simulink model "aeb_rzr"  (R2023b)
settings: Solver=FixedStepAuto  StartTime=0.0  StopTime=inf  RelTol=1e-3
undefined symbols (not defined in the file): camera, gray
libraries: visionanalysis x1, visiongeotforms x1
CloseFcn:
  | helperSLVisionVehicleDetectorCleanUp
settings Model: SILPILSystemUnderTest=refmodels  Creator=The MathWorks, Inc.  LastModifiedBy=tsamak
settings SolverCC: AlgebraicLoopSolver=TrustRegion  MaxZcPerStep=1
settings DataIOCC: SaveFormat=StructureWithTime  SaveOutput=off  DSMLogging=off  SaveTime=off
settings OptimizationCC: DefaultParameterBehavior=Inlined  EnhancedBackFolding=on  PassReuseOutputArgsThreshold=0  ZeroExternalMemoryAtStartup=off  ZeroInternalMemoryAtStartup=off  InitFltsAndDblsToZero=on  OptimizeBlockOrder=speed  DifferentSizesBufferReuse=on  OptimizationCustomize=off
settings DebuggingCC: ParameterTunabilityLossMsg=error  UnconnectedInputMsg=warning  UnconnectedOutputMsg=warning  UnconnectedLineMsg=warning  SubsystemReferenceDiagnosticForUnitTest=warning
settings HardwareCC: ProdLongLongMode=on  TargetLongLongMode=on
settings ModelReferenceCC: EnableRefExpFcnMdlSchedulingChecks=on
settings SFSimCC: SimTargetLang=C++
settings RTWCC: CodeExecutionProfiling=on  CodeProfilingSaveOptions=AllData  TargetLang=C++  GenerateGPUCode=CUDA  DLArmComputeVersion=19.05
settings CodeAppCC: ForceParamTrailComments=on  OperatorAnnotations=on
settings GRTTargetCC: TargetLangStandard=C++11 (ISO)  CodeInterfacePackaging=C++ class
settings ConfigComp: CovScope=ReferencedModels  CovIncludeTopModel=off  CovExternalEMLEnable=off  CovSFcnEnable=off

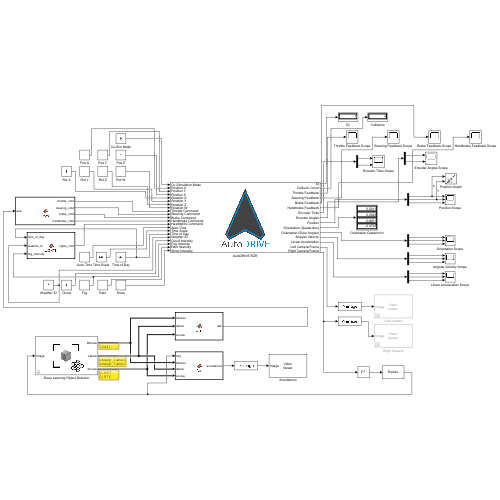
[thumbnail: Simulink's stored preview of the top-level diagram]
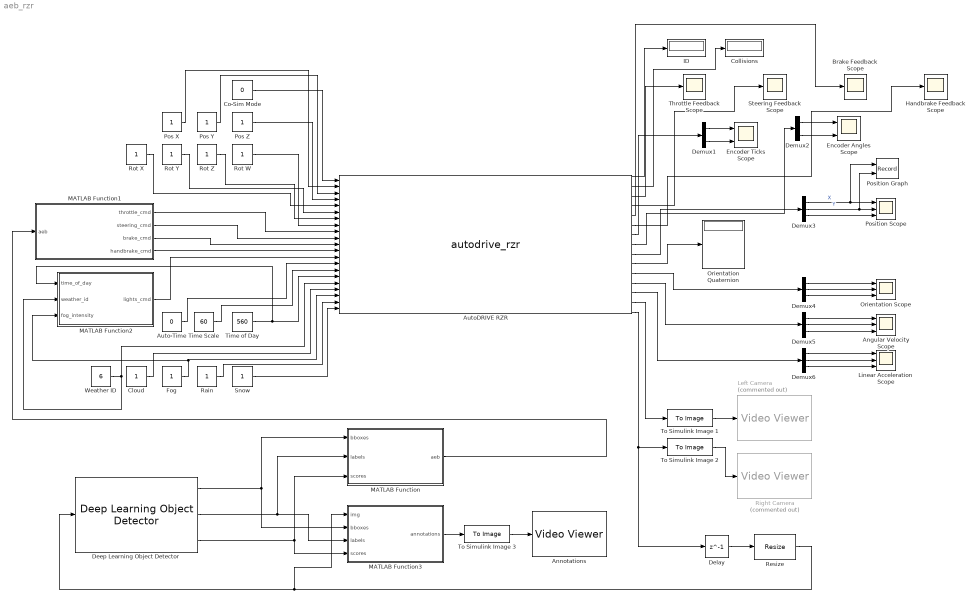
== system aeb_rzr ==
  Angular Velocity Scope : Scope  NumInputPorts=3
  Annotations : VideoViewer  colormapValue=gray(256)  FigPos=[1241.66666666667 442 408 253.333333333333]
  Auto-Time : Constant  Value=0  OutDataTypeStr=boolean
  AutoDRIVE RZR : M-S-Function  FunctionName=autodrive_rzr  Parameters=Port  mask{Port=4567}
      mask Display:
      | image('autodrive_logo.png');
      | port_label('input', 1, 'Co-Simulation Mode');
      | port_label('input', 2, 'Position X');
      | port_label('input', 3, 'Position Y');
      | port_label('input', 4, 'Position Z');
      | port_label('input', 5, 'Rotation X');
      | port_label('input', 6, 'Rotation Y');
      | port_label('input', 7, 'Rotation Z');
      | port_label('input', 8, 'Rotation W');
      | port_label('input', 9, 'Throttle Command');
      | port_label('input', 10, 'Steering Command');
      | port_label('input', 11, 'Brake Command');
      | port_label('input', 12, 'Handbrake Command');
      | port_label('input', 13, 'Headlights Command');
      | port_label('input', 14, 'Auto-Time');
      | port_label('input', 15, 'Time Scale');
      | port_label('input', 16, 'Time of Day');
      | port_label('input', 17, 'Weather ID');
      | port_label('input', 18, 'Cloud Intensity');
      | port_label('input', 19, 'Fog Intensity');
      | port_label('input', 20, 'Rain Intensity');
      | port_label('input', 21, 'Snow Intensity');
      | port_label('output', 1, 'ID');
      | port_label('output', 2, 'Collision Count');
      | port_label('output', 3, 'Throttle Feedback');
      | port_label('output', 4, 'Steering Feedback');
      | port_label('output', 5, 'Brake Feedback');
      | port_label('output', 6, 'Handbrake Feedback');
      | port_label('output', 7, 'Encoder Ticks');
      | port_label('output', 8, 'Encoder Angles');
      | port_label('output', 9, 'Position');
      | port_label('output', 10, 'Orientation (Quaternion)');
      | port_label('output', 11, 'Orientation (Euler Angles)');
      | port_label('output', 12, 'Angular Velocity');
      | port_label('output', 13, 'Linear Acceleration');
      | port_label('output', 14, 'Left Camera Frame');
      | port_label('output', 15, 'Right Camera Frame');
  Brake Feedback Scope : Scope
  Cloud : Constant
  Co-Sim Mode : Constant  Value=0  OutDataTypeStr=uint8
  Collisions : Display
  Deep Learning Object Detector : visionanalysis/Deep Learning Object Detector  Detector=Detector from MAT-file  DetectorFunction=vehicleDetectorYOLOv2  DetectorFilePath=C:\Users\tsamak\Downloads\MathWorks RZR AEB\yolov4_tiny.mat  MaxDetections=10  Bboxes=on  Scores=on  UseROI=off  ROI=[1 1 camera.ImageSize(2) round(camera.ImageSize(1)*0.678)]  Threshold=0.4  NumStrongestRegions=2000  UseMinSize=off  MinSize=[1 1]  UseMaxSize=off  MaxSize=[50 50]  ForceInterpretedSim=off
  Delay : Delay  DelayLength=1
  Demux1 : Demux  Outputs=2
  Demux2 : Demux  Outputs=2
  Demux{3..6} (4 alike) : Demux  Outputs=3
  Encoder Angles Scope : Scope  NumInputPorts=2
  Encoder Ticks Scope : Scope  NumInputPorts=2
  Fog : Constant
  Handbrake Feedback Scope : Scope
  ID : Display
  Left Camera : VideoViewer  Commented=on  colormapValue=gray(256)  FigPos=[11 410 408 304]
  Linear Acceleration Scope : Scope  NumInputPorts=3
  MATLAB Function : MATLAB Function  TreatAsAtomicUnit=on
  MATLAB Function1 : MATLAB Function  TreatAsAtomicUnit=on
  MATLAB Function2 : MATLAB Function  TreatAsAtomicUnit=on
  MATLAB Function3 : MATLAB Function  TreatAsAtomicUnit=on
  Orientation Quaternion : Display
  Orientation Scope : Scope  NumInputPorts=3
  Pos X : Constant
  Pos Y : Constant
  Pos Z : Constant
  Position Graph : Record  FileSettingsInternal="{\"entries\":[{\"content\":{\"excelSettings\":{\"content\":{},\"type\":\"Streamout.ExcelSettings\"}},\"type\":\"Streamout.FileSettingStorage\",\"uuid\":\"\"}],\"packageUris\":[\"http:\\/\\/schema.mathworks.com\\/mf0\\/streamout_blocks\\/R2020a\"],\"version\":\"1.0\"}"  Layout=[1 1]  SignalsInternal="{\"entries\":[{\"content\":{\"signals\":[{\"content\":{\"blockPath\":[],\"dimensions\":[1,1],\"domain\":\"\",\"lineColor\":\"#139fff\",\"plots\":[ 1 ],\"port\":1,\"signalID\":1,\"signalName\":\"X\"},\"type\":\"RecordBlkView.Signal\",\"uuid\":\"\"},{\"content\":{\"blockPath\":[],\"dimensions\":[1,1],\"domain\":\"\",\"lineColor\":\"#139fff\",\"plots\":[ 1 ],\"port\":2,\"signalID\":2,\"signalName\":\"Y\"},\"type\":\"RecordBlkView.Signal\",\"uuid\":\"\"}]},\"type\":\"RecordBlkView.InputSignals\",\"uuid\":\"\"}],\"packageUris\":[\"http:\\/\\/schema.mathworks.com\\/mf0\\/streamout_blocks\\/R2020a\"],\"version\":\"1.0\"}"  VisualizationBindings="{\"xyplotplugin\":{\"info\":[{\"series\":[{\"bindingParametersList\":[{\"parameter\":\"X-Axis\",\"signalID\":1,\"signalName\":\"X\"},{\"parameter\":\"Y-Axis\",\"signalID\":2,\"signalName\":\"Y\"}],\"seriesID\":0}],\"subplotID\":1}]}}"  CompatibilityTag=XY
  Position Scope : Scope  NumInputPorts=3
  Rain : Constant
  Resize : visiongeotforms/Resize  specify=Number of output rows and columns  rfactor=[200 150]  outCols=25  outRows=25  outRowsCols=[360 640]  interp_method=Bilinear  antialias=on  useROI=off  roiFlag=off  roundingMode=Nearest  overflowMode=on  prodOutputMode=Binary point scaling  prodOutputWordLength=32  prodOutputFracLength=10
  Right Camera : VideoViewer  Commented=on  colormapValue=gray(256)  FigPos=[2.33333333333333 406.666666666667 418 304]
  Rot W : Constant
  Rot X : Constant
  Rot Y : Constant
  Rot Z : Constant
  Snow : Constant
  Steering Feedback Scope : Scope
  Throttle Feedback Scope : Scope
  Time Scale : Constant  Value=60
  Time of Day : Constant  Value=560
  To Simulink Image 1 : ToImage
  To Simulink Image 2 : ToImage
  To Simulink Image 3 : ToImage
  Weather ID : Constant  Value=6  OutDataTypeStr=uint8
  wires:
  Demux4/2 -> Orientation Scope/2
  AutoDRIVE RZR/15 -> Delay/1, To Simulink Image 2/1
  AutoDRIVE RZR/2 -> Collisions/1
  MATLAB Function2/1(lights_cmd) -> AutoDRIVE RZR/13
  Pos X/1 -> AutoDRIVE RZR/2
  AutoDRIVE RZR/5 -> Brake Feedback Scope/1
  Snow/1 -> AutoDRIVE RZR/21
  Demux6/2 -> Linear Acceleration Scope/2
  Time Scale/1 -> AutoDRIVE RZR/15
  Fog/1 -> MATLAB Function2/3(fog_intensity), AutoDRIVE RZR/19
  Rot Z/1 -> AutoDRIVE RZR/7
  Demux4/3 -> Orientation Scope/3
  Demux1/2 -> Encoder Ticks Scope/2
  Demux2/2 -> Encoder Angles Scope/2
  AutoDRIVE RZR/8 -> Demux2/1
  Demux5/2 -> Angular Velocity Scope/2
  Pos Y/1 -> AutoDRIVE RZR/3
  Rot Y/1 -> AutoDRIVE RZR/6
  Pos Z/1 -> AutoDRIVE RZR/4
  Demux2/1 -> Encoder Angles Scope/1
  Rot W/1 -> AutoDRIVE RZR/8
  AutoDRIVE RZR/13 -> Demux6/1
  AutoDRIVE RZR/12 -> Demux5/1
  AutoDRIVE RZR/14 -> To Simulink Image 1/1
  AutoDRIVE RZR/11 -> Demux4/1
  Rot X/1 -> AutoDRIVE RZR/5
  AutoDRIVE RZR/3 -> Throttle Feedback Scope/1
  To Simulink Image 1/1 -> Left Camera/1
  Demux3/3 -> Position Scope/3
  Weather ID/1 -> MATLAB Function2/2(weather_id), AutoDRIVE RZR/17
  AutoDRIVE RZR/4 -> Steering Feedback Scope/1
  Demux6/3 -> Linear Acceleration Scope/3
  AutoDRIVE RZR/1 -> ID/1
  Demux3/1 -> Position Scope/1, Position Graph/1  "X"
  To Simulink Image 2/1 -> Right Camera/1
  Demux3/2 -> Position Scope/2, Position Graph/2  "Y"
  Co-Sim Mode/1 -> AutoDRIVE RZR/1
  Demux6/1 -> Linear Acceleration Scope/1
  Demux5/3 -> Angular Velocity Scope/3
  Cloud/1 -> AutoDRIVE RZR/18
  Rain/1 -> AutoDRIVE RZR/20
  Time of Day/1 -> MATLAB Function2/1(time_of_day), AutoDRIVE RZR/16
  AutoDRIVE RZR/10 -> Orientation Quaternion/1
  AutoDRIVE RZR/6 -> Handbrake Feedback Scope/1
  AutoDRIVE RZR/7 -> Demux1/1
  AutoDRIVE RZR/9 -> Demux3/1
  Demux4/1 -> Orientation Scope/1
  Demux5/1 -> Angular Velocity Scope/1
  Auto-Time/1 -> AutoDRIVE RZR/14
  Demux1/1 -> Encoder Ticks Scope/1
  Deep Learning Object Detector/1 -> MATLAB Function3/2(bboxes), MATLAB Function/1(bboxes)
  Deep Learning Object Detector/3 -> MATLAB Function/3(scores), MATLAB Function3/4(scores)
  Deep Learning Object Detector/2 -> MATLAB Function3/3(labels), MATLAB Function/2(labels)
  Resize/1 -> MATLAB Function3/1(img), Deep Learning Object Detector/1
  MATLAB Function/1(aeb) -> MATLAB Function1/1(aeb)
  MATLAB Function1/1(throttle_cmd) -> AutoDRIVE RZR/9
  MATLAB Function1/2(steering_cmd) -> AutoDRIVE RZR/10
  MATLAB Function1/3(brake_cmd) -> AutoDRIVE RZR/11
  MATLAB Function1/4(handbrake_cmd) -> AutoDRIVE RZR/12
  Delay/1 -> Resize/1
  MATLAB Function3/1(annotations) -> To Simulink Image 3/1
  To Simulink Image 3/1 -> Annotations/1

== matlab function aeb_rzr/MATLAB Function ==
  data: bboxes input; aeb output; labels input; scores input
function aeb = AEB(bboxes, labels, scores)
    aeb = 0;
    valid_labels = [yolov4_tiny_labels.bird_label, yolov4_tiny_labels.cat_label, ...
                    yolov4_tiny_labels.dog_label, yolov4_tiny_labels.horse_label, ...
                    yolov4_tiny_labels.sheep_label, yolov4_tiny_labels.cow_label, ...
                    yolov4_tiny_labels.elephant_label, yolov4_tiny_labels.bear_label, ...
                    yolov4_tiny_labels.zebra_label, yolov4_tiny_labels.giraffe_label];
    for i=1:size(bboxes,1)
        if (any(valid_labels(:) == labels(i)))
            if (scores(i) >= 0.5)
                if (bboxes(i,3)*bboxes(i,4) >= 4000)
                    aeb = 1;
                else
                    aeb = 0;
                end
            else
                aeb = 0;
            end
        else
            aeb = 0;
        end
    end

== matlab function aeb_rzr/MATLAB Function1 ==
  data: aeb input; throttle_cmd output; steering_cmd output; brake_cmd output; handbrake_cmd output
function [throttle_cmd,steering_cmd,brake_cmd,handbrake_cmd] = DBW(aeb)
    if (aeb==1)
        throttle_cmd=0;
        steering_cmd=0;
        brake_cmd=1;
        handbrake_cmd=0;
    else
        throttle_cmd=0.25;
        steering_cmd=0;
        brake_cmd=0;
        handbrake_cmd=0;
    end

== matlab function aeb_rzr/MATLAB Function2 ==
  data: time_of_day input; lights_cmd output; weather_id input; fog_intensity input
function lights_cmd  = LIGHTS(time_of_day,weather_id,fog_intensity)
    if (((0 <= time_of_day) && (time_of_day <= 420)) || ((1080 <= time_of_day) && (time_of_day <= 1440))) % Night
        if (weather_id~=1 || weather_id~=2 || (weather_id==0 && fog_intensity ~= 0)) % Foggy night
            lights_cmd = uint8(3); % Vehicle headlights command [0 = Disabled, 1 = Enabled, 2 = Signature Lights, 3 = 1+2]
        else % Clear night
            lights_cmd = uint8(3); % Vehicle headlights command [0 = Disabled, 1 = Enabled, 2 = Signature Lights, 3 = 1+2]
        end
    elseif (weather_id~=1 || weather_id~=2 || (weather_id==0 && fog_intensity ~= 0)) % Foggy day
        lights_cmd = uint8(2); % Vehicle headlights command [0 = Disabled, 1 = Enabled, 2 = Signature Lights, 3 = 1+2]
    else % Clear day
        lights_cmd = uint8(2); % Vehicle headlights command [0 = Disabled, 1 = Enabled, 2 = Signature Lights, 3 = 1+2]
    end

== matlab function aeb_rzr/MATLAB Function3 ==
  data: img input; annotations output; bboxes input; labels input; scores input
function annotations = ANNOTATE(img, bboxes, labels, scores)
    annotations = uint8(zeros(360,640,3));
    annotations = insertObjectAnnotation(img,"rectangle",bboxes,labels);
